simulink model "TenueModale"  (R2019a)
settings: Solver=VariableStepAuto  StartTime=0.0  StopTime=10.0  RelTol=1e-3
values from neighbouring files (symbols this model uses):
  A6 = Acm(iVa:end, iVa:end)    [mainProjetCADV_2a.m]
  B6 = Bcm(iVa:end)    [mainProjetCADV_2a.m]
  C6 = Ccm(iVa:end, iVa:end)    [mainProjetCADV_2a.m]
  DEG2RAD = pi/180.    (= 0.0174532925199)    [mainProjetCADV_2a.m]    (also in utAcDynamicsFunction.m; utConstantAeroCoeff.m)
  H = -inv(C6_pour_h*inv(A6-B6*K6)*B6)    [mainProjetCADV_2a.m]
  K6 = place(A6,B6,[dp, conj(dp), -3.3965 + 0.1541i, -3.3965 - 0.1541i, -5, -6])    [mainProjetCADV_2a.m]
settings Model: Creator=ulyss  LastModifiedBy=ulyss

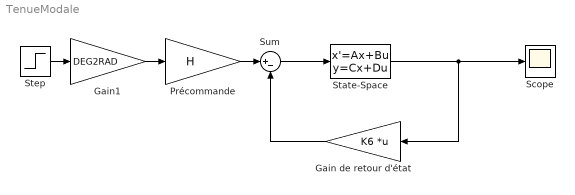
== system TenueModale ==
  Gain de retour d'état : Gain  Gain=K6  Multiplication=Matrix(K*u) (u vector)
  Gain1 : Gain  Gain=DEG2RAD
  Précommande : Gain  Gain=H
  Scope : Scope
  State-Space : StateSpace  A=A6  B=B6  C=C6  D=zeros(6,1)  InitialCondition=0
  Step : Step  After=5  SampleTime=0
  Sum : Sum  Inputs=|+-
  wires:
  Step/1 -> Gain1/1
  Sum/1 -> State-Space/1
  State-Space/1 -> Scope/1, Gain de retour d'état/1
  Gain de retour d'état/1 -> Sum/2
  Gain1/1 -> Précommande/1
  Précommande/1 -> Sum/1
